simulink model "schemat_lab2"  (R2019b)
settings: Solver=ode45  StartTime=0.0  StopTime=100  RelTol=1e-3  AbsTol=1e-6  EnableMultiTasking=on
values from neighbouring files (symbols this model uses):
  cpw = 4175    [LAB1.m]    (also in LAB2.m; LAB3.m)
  Cvg = cpw * row * Vg    (= 40080000)    [LAB1.m]    (also in LAB2.m; bezp.m = 832608.1632; budynek_z_hydraulika_symulacja.m = 999129.79584; grzejnik_pi_skrypt.m = 83260.81632)
  Cvk = Cvg    (= 40080000)    [LAB2.m]    (also in LAB3.m = 4175000; bezp.m = 4163040.816; budynek_z_hydraulika_symulacja.m = 249782.44896; kociol_pokoj_skrypt.m = 4163040.816)
  Cvw = cpp * rop * Vp    (= 108000)    [LAB1.m]    (also in LAB2.m; bezp.m = 870775.92; budynek_z_hydraulika_symulacja.m = 83613.6; grzejnik_pi_skrypt.m = 83613.6)
  dfmg = 0    [LAB1.m]    (also in LAB2.m)
  dfmk = 0    [LAB2.m]    (also in LAB3.m)
  dqk = 0    [LAB2.m]    (also in LAB3.m = 2200)
  dTzew = 0    [LAB1.m]    (also in LAB2.m; bezp.m; budynek_z_hydraulika_symulacja.m; grzejnik_pi_skrypt.m)
  fmgN = qgN/(TgzN-TgpN)    (= 1000)    [LAB1.m]    (also in LAB2.m)
  fmk0 = fmkN    (= 1000)    [LAB2.m]    (also in LAB3.m = 0.131736526946)
  Kcg = qgN/(TgpN - TwewN)    (= 400)    [LAB1.m]    (also in LAB2.m)
  Kcw = qgN/(TwewN-TzewN)    (= 500)    [LAB1.m]    (also in LAB2.m)
  qk0 = qgN    (= 20000)    [LAB2.m]    (also in LAB3.m = 11000)
  TgpN = 70    [LAB1.m]    (also in LAB2.m)
  TwewN = 20    [LAB1.m]    (also in LAB2.m)
  Tzew0 = TzewN    (= -20)    [LAB1.m]    (also in LAB2.m; LAB3.m; bezp.m = -13; grzejnik_pi_skrypt.m)
settings Model: Creator=LAB320-1552  LastModifiedBy=LAB320
settings SolverCC: AutoScaleAbsTol=off
settings DataIOCC: LimitDataPoints=on  SaveFormat=Array  ReturnWorkspaceOutputs=off
settings OptimizationCC: LifeSpan=inf
settings DebuggingCC: UnderspecifiedInitializationDetection=Classic  MergeDetectMultiDrivingBlocksExec=none  StateNameClashWarn=warning  SFUnexpectedBacktrackingDiag=warning  SFNoUnconditionalDefaultTransitionDiag=warning  SFExecutionAtInitializationDiag=none  ArithmeticOperatorsInVariantConditions=warning
settings HardwareCC: ProdBitPerPointer=32  ProdBitPerSizeT=32  ProdBitPerPtrDiffT=32  ProdLargestAtomicFloat=None  ProdIntDivRoundTo=Undefined  ProdEndianess=Unspecified  ProdWordSize=32  ProdHWDeviceType=32-bit Generic
settings ModelReferenceCC: PropagateSignalLabelsOutOfModel=off
settings SFSimCC: SimUseLocalCustomCode=off  CustomCodeUndefinedFunction=UseInterfaceOnly
settings RTWCC: RTWUseLocalCustomCode=off
settings CodeAppCC: StateflowObjectComments=on
settings GRTTargetCC: TargetLangStandard=C89/C90 (ANSI)  GeneratePreprocessorConditionals=Disable all
settings ConfigComp: CovMetricSettings=dw  CovHtmlReporting=on  CovSaveCumulativeToWorkspaceVar=on  CovSaveSingleToWorkspaceVar=on  CovExternalEMLEnable=off

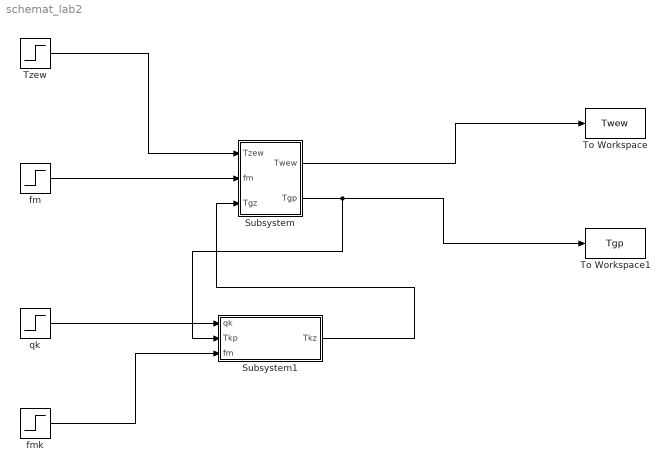
== system schemat_lab2 ==
  Subsystem : Subsystem  mask{Kcw=Kcw, Kcg=Kcg, Cvw=Cvw, Cvg=Cvg}
  Subsystem1 : Subsystem  mask{cpw=cpw, Cvk=Cvk}
  To Workspace : ToWorkspace  VariableName=Twew  SampleTime=-1
  To Workspace1 : ToWorkspace  VariableName=Tgp  SampleTime=-1
  "Tzew " : Step  Before=Tzew0 + dTzew  After=Tzew0 + dTzew  SampleTime=0
  "fm " : Step  Before=fmgN + dfmg  After=fmgN + dfmg  SampleTime=0
  fmk : Step  Before=fmk0 + dfmk  After=fmk0 + dfmk  SampleTime=0
  qk : Step  Before=qk0 + dqk  After=qk0 + dqk  SampleTime=0
  wires:
  "Tzew "/1 -> Subsystem/1(Tzew)
  "fm "/1 -> Subsystem/2(fm)
  Subsystem/1(Twew) -> To Workspace/1
  Subsystem/2(Tgp) -> Subsystem1/2(Tkp), To Workspace1/1
  qk/1 -> Subsystem1/1(qk)
  Subsystem1/1(Tkz) -> Subsystem/3(Tgz)
  fmk/1 -> Subsystem1/3(fm)

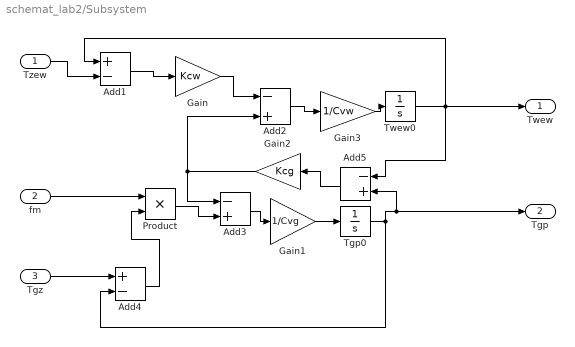
== system schemat_lab2/Subsystem ==
  Tzew : Inport
  fm : Inport  Port=2
  Tgz : Inport  Port=3
  Add1 : Sum  Inputs=+-
  Add2 : Sum  Inputs=-+
  Add3 : Sum  Inputs=-+
  Add4 : Sum  Inputs=+-
  Add5 : Sum  Inputs=-+
  Gain : Gain  Gain=Kcw
  Gain1 : Gain  Gain=1/Cvg
  Gain2 : Gain  Gain=Kcg
  Gain3 : Gain  Gain=1/Cvw
  Product : Product
  Tgp0 : Integrator  InitialCondition=TgpN
  Twew0 : Integrator  InitialCondition=TwewN
  Twew : Outport
  Tgp : Outport  Port=2
  wires:
  Product/1 -> Add3/2
  Tgz/1 -> Add4/1
  Gain/1 -> Add2/1
  Add2/1 -> Gain3/1
  Add4/1 -> Product/2
  Add1/1 -> Gain/1
  Gain2/1 -> Add2/2, Add3/1
  Twew0/1 -> Twew/1, Add1/1, Add5/1
  Gain1/1 -> Tgp0/1
  Tgp0/1 -> Tgp/1, Add5/2, Add4/2
  Add3/1 -> Gain1/1
  Add5/1 -> Gain2/1
  Gain3/1 -> Twew0/1
  Tzew/1 -> Add1/2
  fm/1 -> Product/1

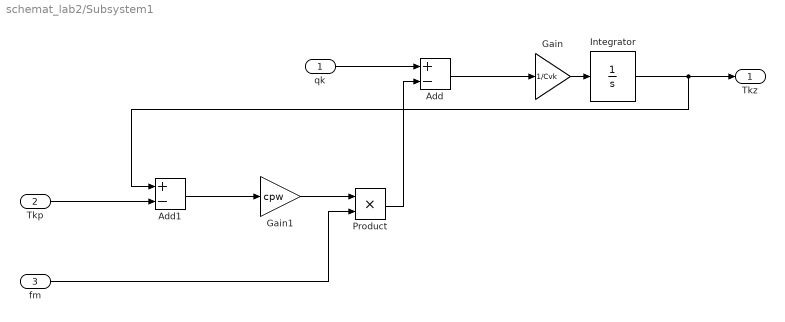
== system schemat_lab2/Subsystem1 ==
  qk : Inport
  Tkp : Inport  Port=2
  fm : Inport  Port=3
  Add : Sum  Inputs=+-
  Add1 : Sum  Inputs=+-
  Gain : Gain  Gain=1/Cvk
  Gain1 : Gain  Gain=cpw
  Integrator : Integrator
  Product : Product
  Tkz : Outport
  wires:
  Gain/1 -> Integrator/1
  qk/1 -> Add/1
  Add/1 -> Gain/1
  Tkp/1 -> Add1/2
  Integrator/1 -> Add1/1, Tkz/1
  Add1/1 -> Gain1/1
  fm/1 -> Product/2
  Gain1/1 -> Product/1
  Product/1 -> Add/2
